simulink model "Single_Axis_Yaw_Disturbance"  (R2024b)
settings: Solver=ode4  StartTime=0.0  StopTime=0.2  FixedStep=0.001  RelTol=1e-3
settings Model: Creator=Zohaib  LastModifiedBy=Zohaib
settings DataIOCC: ReturnWorkspaceOutputs=off

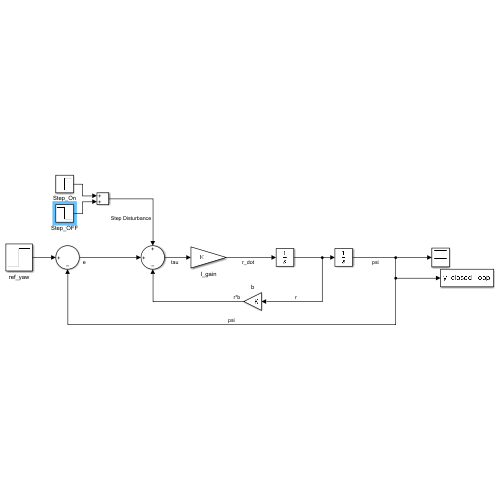
[thumbnail: Simulink's stored preview of the top-level diagram]
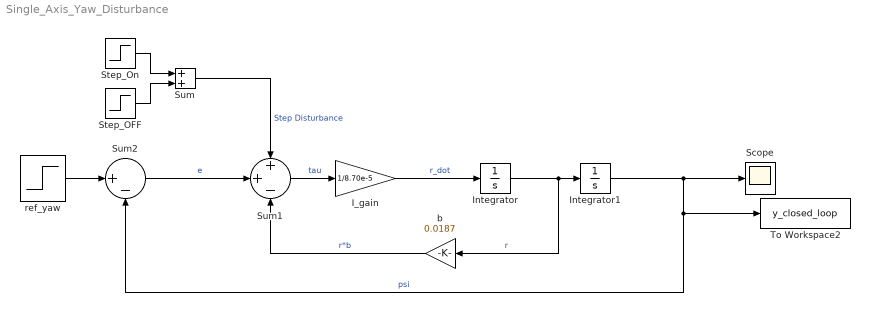
== system Single_Axis_Yaw_Disturbance ==
  I_gain : Gain  Gain=1/8.70e-5
  Integrator : Integrator
  Integrator1 : Integrator
  Scope : Scope
  Step_OFF : Step  Time=0.1235  After=-0.001  SampleTime=0.001
  Step_On : Step  Time=0.12  After=0.001  SampleTime=0.001
  Sum : Sum
  Sum1 : Sum  Inputs=++-
  Sum2 : Sum  Inputs=|+-
  To Workspace2 : ToWorkspace  VariableName=y_closed_loop  SaveFormat=Timeseries  SampleTime=-1
  b : Gain  Gain=0.0187
  ref_yaw : Step  Time=0  After=5*(pi/180)  SampleTime=0.001
  wires:
  Integrator1/1 -> Sum2/2, To Workspace2/1, Scope/1  "psi"
  Integrator/1 -> b/1, Integrator1/1  "r"
  Sum1/1 -> I_gain/1  "tau"
  I_gain/1 -> Integrator/1  "r_dot"
  ref_yaw/1 -> Sum2/1
  Step_On/1 -> Sum/1
  Step_OFF/1 -> Sum/2
  b/1 -> Sum1/3  "r*b"
  Sum2/1 -> Sum1/2  "e"
  Sum/1 -> Sum1/1  "Step Disturbance"
